simulink model "SF051A_SnsrOffsLrng"  (R2013b)
settings: Solver=FixedStepDiscrete  SolverMode=SingleTasking  StartTime=0.0  StopTime=1  FixedStep=0.002  RelTol=1e-3
values from neighbouring files (symbols this model uses):
  ARCHGLBPRM_10MILLISEC_SEC_F32 = DataDict.Constant    [SF051A_SnsrOffsLrng_DataDict.m]
  ARCHGLBPRM_2MILLISEC_SEC_F32 = DataDict.Constant    [SF051A_SnsrOffsLrng_DataDict.m]
  ARCHGLBPRM_2PI_ULS_F32 = DataDict.Constant    [SF051A_SnsrOffsLrng_DataDict.m]
  ARCHGLBPRM_FLOATZEROTHD_ULS_F32 = DataDict.Constant    [SF051A_SnsrOffsLrng_DataDict.m]
  ARCHGLBPRM_PIOVER180_ULS_F32 = DataDict.Constant    [SF051A_SnsrOffsLrng_DataDict.m]
  CNV100MICROSECTOSEC_SECPERCNT_F32 = DataDict.Constant    [SF051A_SnsrOffsLrng_DataDict.m]
  COVRAMTRXNIT_ULS_F32 = DataDict.Constant    [SF051A_SnsrOffsLrng_DataDict.m]
  HWAGHILIM_HWDEG_F32 = DataDict.Constant    [SF051A_SnsrOffsLrng_DataDict.m]
  HWAUTHYTHD_ULS_F32 = DataDict.Constant    [SF051A_SnsrOffsLrng_DataDict.m]
  HWTQLRNGSTSLRND_CNT_U08 = DataDict.Constant    [SF051A_SnsrOffsLrng_DataDict.m]
  HWTQLRNGSTSNEGOFFS_CNT_U08 = DataDict.Constant    [SF051A_SnsrOffsLrng_DataDict.m]
  HWTQLRNGSTSNOTLRND_CNT_U08 = DataDict.Constant    [SF051A_SnsrOffsLrng_DataDict.m]
  HWTQLRNGSTSPOSOFFS_CNT_U08 = DataDict.Constant    [SF051A_SnsrOffsLrng_DataDict.m]
  HWTQLRNGSTSZEROOFFS_CNT_U08 = DataDict.Constant    [SF051A_SnsrOffsLrng_DataDict.m]
  IDYMTRX_ULS_F32 = DataDict.Constant    [SF051A_SnsrOffsLrng_DataDict.m]
  IVS10MS_ULSPERSEC_F32 = DataDict.Constant    [SF051A_SnsrOffsLrng_DataDict.m]
  LRNGFILTICON_ULS_F32 = DataDict.Constant    [SF051A_SnsrOffsLrng_DataDict.m]
  ONE_ULS_F32 = DataDict.Constant    [SF051A_SnsrOffsLrng_DataDict.m]
  SnsrOffsLrnd = DataDict.NVM    [SF051A_SnsrOffsLrng_DataDict.m]
  SnsrOffsLrngFctEna = DataDict.Calibration    [SF051A_SnsrOffsLrng_DataDict.m]
  SnsrOffsLrngHwAgLrngDrvgDstThd = DataDict.Calibration    [SF051A_SnsrOffsLrng_DataDict.m]
  SnsrOffsLrngHwAgLrngEna = DataDict.Calibration    [SF051A_SnsrOffsLrng_DataDict.m]
  SnsrOffsLrngHwAgLrngHwVelThd = DataDict.Calibration    [SF051A_SnsrOffsLrng_DataDict.m]
  SnsrOffsLrngHwAgLrngSysTqThd = DataDict.Calibration    [SF051A_SnsrOffsLrng_DataDict.m]
  SnsrOffsLrngHwAgLrngSysTqThdMed = DataDict.Calibration    [SF051A_SnsrOffsLrng_DataDict.m]
  SnsrOffsLrngHwAgLrngSysTqThdTrustd = DataDict.Calibration    [SF051A_SnsrOffsLrng_DataDict.m]
  SnsrOffsLrngHwAgLrngSysTqThdWide = DataDict.Calibration    [SF051A_SnsrOffsLrng_DataDict.m]
  SnsrOffsLrngHwAgLrngTi = DataDict.Calibration    [SF051A_SnsrOffsLrng_DataDict.m]
  SnsrOffsLrngHwAgLrngVehSpdThd = DataDict.Calibration    [SF051A_SnsrOffsLrng_DataDict.m]
  SnsrOffsLrngHwAgLrngYawOffsDbnd = DataDict.Calibration    [SF051A_SnsrOffsLrng_DataDict.m]
  SnsrOffsLrngHwAgLrngYawRateThd = DataDict.Calibration    [SF051A_SnsrOffsLrng_DataDict.m]
  SnsrOffsLrngHwAgOffsLim = DataDict.Calibration    [SF051A_SnsrOffsLrng_DataDict.m]
  SnsrOffsLrngHwTqLrngEna = DataDict.Calibration    [SF051A_SnsrOffsLrng_DataDict.m]
  SnsrOffsLrngHwTqLrngEnaTiThd = DataDict.Calibration    [SF051A_SnsrOffsLrng_DataDict.m]
  SnsrOffsLrngHwTqLrngHwAgDbnd = DataDict.Calibration    [SF051A_SnsrOffsLrng_DataDict.m]
  SnsrOffsLrngHwTqLrngHwAgThd = DataDict.Calibration    [SF051A_SnsrOffsLrng_DataDict.m]
  SnsrOffsLrngHwTqLrngHwTqThd = DataDict.Calibration    [SF051A_SnsrOffsLrng_DataDict.m]
  SnsrOffsLrngHwTqLrngHwTqZeroOffsThd = DataDict.Calibration    [SF051A_SnsrOffsLrng_DataDict.m]
  SnsrOffsLrngHwTqLrngHwVelThd = DataDict.Calibration    [SF051A_SnsrOffsLrng_DataDict.m]
  SnsrOffsLrngHwTqLrngMeasTi = DataDict.Calibration    [SF051A_SnsrOffsLrng_DataDict.m]
  SnsrOffsLrngHwTqLrngMeasTiScar = DataDict.Calibration    [SF051A_SnsrOffsLrng_DataDict.m]
  SnsrOffsLrngHwTqLrngSampleImbThd1 = DataDict.Calibration    [SF051A_SnsrOffsLrng_DataDict.m]
  SnsrOffsLrngHwTqLrngSampleImbThd2 = DataDict.Calibration    [SF051A_SnsrOffsLrng_DataDict.m]
  SnsrOffsLrngHwTqLrngSampleThd1 = DataDict.Calibration    [SF051A_SnsrOffsLrng_DataDict.m]
  SnsrOffsLrngHwTqLrngSampleThd2 = DataDict.Calibration    [SF051A_SnsrOffsLrng_DataDict.m]
  SnsrOffsLrngHwTqLrngTiWghtCoeff = DataDict.Calibration    [SF051A_SnsrOffsLrng_DataDict.m]
  SnsrOffsLrngHwTqLrngVehSpdThd = DataDict.Calibration    [SF051A_SnsrOffsLrng_DataDict.m]
  SnsrOffsLrngHwTqOffsLim = DataDict.Calibration    [SF051A_SnsrOffsLrng_DataDict.m]
  SnsrOffsLrngSampleCntForHwTqLrngRst = DataDict.Calibration    [SF051A_SnsrOffsLrng_DataDict.m]
  SnsrOffsLrngTqInpDetnPwrEstimnThd = DataDict.Calibration    [SF051A_SnsrOffsLrng_DataDict.m]
  SnsrOffsLrngTqInpDetnSinGenrAmp = DataDict.Calibration    [SF051A_SnsrOffsLrng_DataDict.m]
  SnsrOffsLrngTqInpDetnSinGenrFrq = DataDict.Calibration    [SF051A_SnsrOffsLrng_DataDict.m]
  SnsrOffsLrngTqInpDetnStg1FilGain = DataDict.Calibration    [SF051A_SnsrOffsLrng_DataDict.m]
  SnsrOffsLrngTqInpDetnStg1WinSize = DataDict.Calibration    [SF051A_SnsrOffsLrng_DataDict.m]
  SnsrOffsLrngTqInpDetnStg2FilGainCen = DataDict.Calibration    [SF051A_SnsrOffsLrng_DataDict.m]
  SnsrOffsLrngTqInpDetnStg2FilGainDwn = DataDict.Calibration    [SF051A_SnsrOffsLrng_DataDict.m]
  SnsrOffsLrngTqInpDetnStg2FilGainUp = DataDict.Calibration    [SF051A_SnsrOffsLrng_DataDict.m]
  SnsrOffsLrngTqInpDetnStg2WinSize = DataDict.Calibration    [SF051A_SnsrOffsLrng_DataDict.m]
  SnsrOffsLrngYawLrngEna = DataDict.Calibration    [SF051A_SnsrOffsLrng_DataDict.m]
  SnsrOffsLrngYawLrngHwAgThd = DataDict.Calibration    [SF051A_SnsrOffsLrng_DataDict.m]
  SnsrOffsLrngYawLrngTi = DataDict.Calibration    [SF051A_SnsrOffsLrng_DataDict.m]
  SnsrOffsLrngYawLrngYawAThd = DataDict.Calibration    [SF051A_SnsrOffsLrng_DataDict.m]
  SnsrOffsLrngYawOffsFrshTiThd = DataDict.Calibration    [SF051A_SnsrOffsLrng_DataDict.m]
  SnsrOffsLrngYawRateOffsLim = DataDict.Calibration    [SF051A_SnsrOffsLrng_DataDict.m]
  SPDCNVN_MTRPERSECPERKPH_F32 = DataDict.Constant    [SF051A_SnsrOffsLrng_DataDict.m]
  SysGlbPrmSysTqRat = DataDict.ImprtdCal    [SF051A_SnsrOffsLrng_DataDict.m]
  TISTEP10MS_MINS_F32 = DataDict.Constant    [SF051A_SnsrOffsLrng_DataDict.m]
  TQINPDETNLOGGAIN_ULS_F32 = DataDict.Constant    [SF051A_SnsrOffsLrng_DataDict.m]
  YAWELPDTIHILIM_MINS_F32 = DataDict.Constant    [SF051A_SnsrOffsLrng_DataDict.m]
  YAWRATENOISE_VEHDEGPERSEC_F32 = DataDict.Constant    [SF051A_SnsrOffsLrng_DataDict.m]
  ZERO_ULS_F32 = DataDict.Constant    [SF051A_SnsrOffsLrng_DataDict.m]
  ZEROVECT_ULS_F32 = DataDict.Constant    [SF051A_SnsrOffsLrng_DataDict.m]
undefined symbols (not defined in the file or in its folder): NvmGetErrSts1
libraries: Fil x34, NxtrLim x20, FixdToFloat x17, FloatToFixd x16, simulink x12, NxtrAbslt x12, NxtrNvM x8, NxtrMath x3
(part 11 of 12)

== system SF051A_SnsrOffsLrng/SnsrOffsLrng/SnsrOffsLrngPer2/Enable_Function/POC/Learn/BiasEstimation_ValidityCheck/HwTqAvrg_Check ==
  note: SysTrq is the addition of the Driver's torque and the Assist torque
      | (in HwNm coordinates)
  note: SysTrqAVG is the average SysTrq during the time that the
      | Learning filters were enabled.
  note: TOCStatus
      | 0 = HwTrq NotLearned
      | 1 = Positive HwTrq Offset
      | 2 = Negative HwTrqOffset
      | 3 = Zero HwTrq Offset
      | 4 = HwTrq Offset Learned
  SysTqAvrg : Inport
  HwTqLrngSts : Inport  Port=2  OutDataTypeStr=uint8
  Constant : Constant  Value=SnsrOffsLrngHwAgLrngSysTqThdTrustd  OutDataTypeStr=single
  Constant1 : Constant  Value=SnsrOffsLrngHwAgLrngSysTqThdWide  OutDataTypeStr=single
  Constant2 : Constant  Value=SnsrOffsLrngHwAgLrngSysTqThdMed  OutDataTypeStr=single
  Display1 : DataStoreWrite  DataStoreName=dSnsrOffsLrngHwAgLrngSysTqUpThd
  Display2 : DataStoreWrite  DataStoreName=dSnsrOffsLrngHwAgLrngSysTqLoThd
  Display3 : DataStoreWrite  DataStoreName=dSnsrOffsLrngHwAgLrngSysTqVldt
  Logical Operator : Logic  AllPortsSameDT=off  OutDataTypeStr=boolean
  Merge_LowTh : Merge  Inputs=6
  Merge_UpTh : Merge  Inputs=6
  Relational Operator : RelationalOperator  Operator=<=  OutDataTypeStr=boolean
  Relational Operator1 : RelationalOperator  OutDataTypeStr=boolean
  Subsystem5 : Subsystem  Description=|  mask(Copyright Information){none=on}
      | Copyright info block.                                               
      |                                                                     
      | Place copyright information at the top of every subsystem in design.
      mask prompts: none "No parameters"
      mask help: Place copyright information at the top of every subsystem in design.
      mask Display:
      | NxtrConf = 'Nexteer Confidential';
      | 
      | sys = bdroot; %handle for the current model ("system")
      | first = get_param(sys,'Created');
      | first = first(end-3:end);  %year is last four digits
      | 
      | last = get_param(sys,'LastModifiedDate');
      | if isempty(last)
      |     last = datestr(now,'yyyy');
      | else
      |     last = last(end-3:end);
      | end
      | 
      | if strcmp(first,last)
      |     fprintf('%s -- Copyright %s Nexteer',NxtrConf,first)
      | else
      |     fprintf('%s -- %s%s- %s Nexteer',NxtrConf,char(169),first,last)
      | end
  Switch Case : SwitchCase  CaseConditions={0,1,2,3,4}
  Switch Case Action Subsystem : Subsystem  RequirementInfo="{'linktype_rmi_doors' '0000babd (/E-STEER Core/SubSystem Specifications/Application Functions/SF051A Sensor Offset Learning)' '#SF051A_146' 'true' 'REQ:  SF051A_146' '' } %GIDa_e88fd376_b621_43d8_82e5_da5b2ad99d04"  TreatAsAtomicUnit=on
  Switch Case Action Subsystem1 : Subsystem  RequirementInfo="{'linktype_rmi_doors' '0000babd (/E-STEER Core/SubSystem Specifications/Application Functions/SF051A Sensor Offset Learning)' '#SF051A_145' 'true' 'REQ:  SF051A_145' '' } %GIDa_07809d37_1ffe_4fb4_b852_393f01c2375c"  TreatAsAtomicUnit=on
  Switch Case Action Subsystem2 : Subsystem  RequirementInfo="{'linktype_rmi_doors' '0000babd (/E-STEER Core/SubSystem Specifications/Application Functions/SF051A Sensor Offset Learning)' '#SF051A_144' 'true' 'REQ:  SF051A_144' '' } %GIDa_dd268c2c_ea11_4446_9a40_dacfc2e25d53"  TreatAsAtomicUnit=on
  Switch Case Action Subsystem3 : Subsystem  RequirementInfo={'linktype_rmi_doors' '0000babd (/E-STEER Core/SubSystem Specifications/Application Functions/SF051A Sensor Offset Learning)' '#SF051A_143' 'true' 'REQ: SF051A_143' '' } %GIDa_217b07df_1d8f_435d_a8bd_62cab7965346  TreatAsAtomicUnit=on
  Switch Case Action Subsystem4 : Subsystem  RequirementInfo="{'linktype_rmi_doors' '0000babd (/E-STEER Core/SubSystem Specifications/Application Functions/SF051A Sensor Offset Learning)' '#SF051A_142' 'true' 'REQ:  SF051A_142' '' } %GIDa_01db2596_4f13_4ac9_b73b_dfc9e16a8861"  TreatAsAtomicUnit=on
  Switch Case Action Subsystem5 : Subsystem  TreatAsAtomicUnit=on
  TqVldFlg : Outport
  wires:
  HwTqLrngSts/1 -> Switch Case/1
  Switch Case Action Subsystem/1(UpTh) -> Merge_UpTh/1
  Merge_UpTh/1 -> Relational Operator/2, Display1/1
  Merge_LowTh/1 -> Display2/1, Relational Operator1/2
  Switch Case/2 -> Switch Case Action Subsystem1/Action
  Switch Case/3 -> Switch Case Action Subsystem2/Action
  Switch Case/4 -> Switch Case Action Subsystem3/Action
  Switch Case/5 -> Switch Case Action Subsystem4/Action
  Switch Case Action Subsystem1/1(UpTh) -> Merge_UpTh/2
  Switch Case Action Subsystem2/1(UpTh) -> Merge_UpTh/3
  Switch Case Action Subsystem3/1(UpTh) -> Merge_UpTh/4
  Switch Case Action Subsystem4/1(UpTh) -> Merge_UpTh/5
  Switch Case Action Subsystem/2(LowTh) -> Merge_LowTh/1
  Switch Case Action Subsystem1/2(LowTh) -> Merge_LowTh/2
  Switch Case Action Subsystem2/2(LowTh) -> Merge_LowTh/3
  Switch Case Action Subsystem3/2(LowTh) -> Merge_LowTh/4
  Switch Case Action Subsystem4/2(LowTh) -> Merge_LowTh/5
  Constant1/1 -> Switch Case Action Subsystem2/1(SysTqThdWide), Switch Case Action Subsystem5/1(SysTqThdWide), Switch Case Action Subsystem1/1(SysTqThdWide), Switch Case Action Subsystem/1(SysTqThdWide)
  Constant/1 -> Switch Case Action Subsystem4/1(SysTqThdTrustd)
  Constant2/1 -> Switch Case Action Subsystem3/1(SysTqThdMed)
  Switch Case/6 -> Switch Case Action Subsystem5/Action
  Switch Case/1 -> Switch Case Action Subsystem/Action
  Switch Case Action Subsystem5/1(UpTh) -> Merge_UpTh/6
  Switch Case Action Subsystem5/2(LowTh) -> Merge_LowTh/6
  SysTqAvrg/1 -> Relational Operator/1, Relational Operator1/1
  Relational Operator/1 -> Logical Operator/1
  Logical Operator/1 -> Display3/1, TqVldFlg/1
  Relational Operator1/1 -> Logical Operator/2

== system SF051A_SnsrOffsLrng/SnsrOffsLrng/SnsrOffsLrngPer2/Enable_Function/POC/Learn/BiasEstimation_ValidityCheck/Limit and Keep Learned Value ==
  HwPosBiasEstRaw : Inport
  Action Port : ActionPort  ActionType=then
  Constant : Constant  RequirementInfo={'linktype_rmi_doors' '0000babd (/E-STEER Core/SubSystem Specifications/Application Functions/SF051A Sensor Offset Learning)' '#SF051A_138' 'true' 'REQ: SF051A_138' '' } %GIDa_21289eda_9e85_4347_9687_653c781a611d  Value=ZERO_ULS_F32  OutDataTypeStr=single
      settings: AttributesFormatString=%<OutDataTypeStr>
  Constant1 : Constant  RequirementInfo="{'linktype_rmi_doors' '0000babd (/E-STEER Core/SubSystem Specifications/Application Functions/SF051A Sensor Offset Learning)' '#SF051A_140' 'true' 'REQ:  SF051A_140' '' } %GIDa_a6f07fad_f17c_4ace_8365_667990c14b30"  Value=SnsrOffsLrngHwAgOffsLim  OutDataTypeStr=single
  FloatToFixd_s16_f32 : FloatToFixd/FloatToFixd_s16_f32  Param1=10
  LimDyn_f32 : NxtrLim/LimDyn_f32  RequirementInfo="{'linktype_rmi_doors' '0000babd (/E-STEER Core/SubSystem Specifications/Application Functions/SF051A Sensor Offset Learning)' '#SF051A_140' 'true' 'REQ:  SF051A_140' '' } %GIDa_2915a7af_cb2e_4592_b132_f2e0d313b25c"
  NVM Ram : DataStoreWrite  RequirementInfo="{'linktype_rmi_doors' '0000babd (/E-STEER Core/SubSystem Specifications/Application Functions/SF051A Sensor Offset Learning)' '#SF051A_120' 'true' 'REQ: SF051A_120' '' ; 'linktype_rmi_doors' '0000babd (/E-STEER Core/SubSystem Specifications/Application Functions/SF051A Sensor Offset Learning)' '#SF051A_119' 'true' 'REQ:  SF051A_119' '' } %GIDa_c18d5963_4a3f_423e_af1b_c67d16260ba6"  DataStoreName=SnsrOffsLrnd  DataStoreElements=SnsrOffsLrnd.HwAgLrndTi#SnsrOffsLrnd.HwAgOffs
  Subsystem5 : Subsystem  Description=|  mask(Copyright Information){none=on}
      | Copyright info block.                                               
      |                                                                     
      | Place copyright information at the top of every subsystem in design.
      mask prompts: none "No parameters"
      mask help: Place copyright information at the top of every subsystem in design.
      mask Display:
      | NxtrConf = 'Nexteer Confidential';
      | 
      | sys = bdroot; %handle for the current model ("system")
      | first = get_param(sys,'Created');
      | first = first(end-3:end);  %year is last four digits
      | 
      | last = get_param(sys,'LastModifiedDate');
      | if isempty(last)
      |     last = datestr(now,'yyyy');
      | else
      |     last = last(end-3:end);
      | end
      | 
      | if strcmp(first,last)
      |     fprintf('%s -- Copyright %s Nexteer',NxtrConf,first)
      | else
      |     fprintf('%s -- %s%s- %s Nexteer',NxtrConf,char(169),first,last)
      | end
  Unary Minus : UnaryMinus  RequirementInfo="{'linktype_rmi_doors' '0000babd (/E-STEER Core/SubSystem Specifications/Application Functions/SF051A Sensor Offset Learning)' '#SF051A_140' 'true' 'REQ:  SF051A_140' '' } %GIDa_fa7a1a43_c58a_4d89_8cd2_8f38148a6033"
  wires:
  Constant/1 -> NVM Ram/1
  LimDyn_f32/1 -> FloatToFixd_s16_f32/1
  Unary Minus/1 -> LimDyn_f32/2
  Constant1/1 -> LimDyn_f32/3, Unary Minus/1
  HwPosBiasEstRaw/1 -> LimDyn_f32/1
  FloatToFixd_s16_f32/1 -> NVM Ram/2

== system SF051A_SnsrOffsLrng/SnsrOffsLrng/SnsrOffsLrngPer2/Enable_Function/POC/Learn/BiasEstimation_ValidityCheck/Reset_HwAgLrng ==
  note: Suggest coding as inline local function: void Reset_HwAg_Learning()
  note: Set HwAg Offlset learning filter back to the last good learned value written to NVM Ram.
      | Set elapsed learning time back to zero.
  note: Reset timer
  note: Reset filters
  Action Port : ActionPort  ActionType=elseif
  Constant : Constant  RequirementInfo="{'linktype_rmi_doors' '0000babd (/E-STEER Core/SubSystem Specifications/Application Functions/SF051A Sensor Offset Learning)' '#SF051A_139' 'true' 'REQ:  SF051A_139' '' } %GIDa_4560022c_466c_4507_b52b_9d9e5f5221da"  Value=ZERO_ULS_F32  OutDataTypeStr=single
      settings: AttributesFormatString=%<OutDataTypeStr>
  Constant1 : Constant  RequirementInfo="{'linktype_rmi_doors' '0000babd (/E-STEER Core/SubSystem Specifications/Application Functions/SF051A Sensor Offset Learning)' '#SF051A_139' 'true' 'REQ:  SF051A_139' '' } %GIDa_5e13df5a_3650_4084_aa1a_80989b1f2780"  Value=ZERO_ULS_F32  OutDataTypeStr=single
      settings: AttributesFormatString=%<OutDataTypeStr>
  Filter SV : DataStoreWrite  RequirementInfo="{'linktype_rmi_doors' '0000babd (/E-STEER Core/SubSystem Specifications/Application Functions/SF051A Sensor Offset Learning)' '#SF051A_139' 'true' 'REQ:  SF051A_139' '' } %GIDa_be755dd9_fcb9_4425_99f4_faf64e25047e"  DataStoreName=HwAgLrngFil1  DataStoreElements=HwAgLrngFil1.FilSt
  Filter SV1 : DataStoreWrite  RequirementInfo="{'linktype_rmi_doors' '0000babd (/E-STEER Core/SubSystem Specifications/Application Functions/SF051A Sensor Offset Learning)' '#SF051A_139' 'true' 'REQ:  SF051A_139' '' } %GIDa_db09f921_4b2f_4c4a_a571_f8085cef7377"  DataStoreName=HwAgLrngFil2  DataStoreElements=HwAgLrngFil2.FilSt
  Filter SV2 : DataStoreWrite  RequirementInfo="{'linktype_rmi_doors' '0000babd (/E-STEER Core/SubSystem Specifications/Application Functions/SF051A Sensor Offset Learning)' '#SF051A_139' 'true' 'REQ:  SF051A_139' '' } %GIDa_eca337dd_6526_4b71_a1b3_c946e62c85db"  DataStoreName=HwAgLrngSysTqFil1  DataStoreElements=HwAgLrngSysTqFil1.FilSt
  Filter SV3 : DataStoreWrite  RequirementInfo="{'linktype_rmi_doors' '0000babd (/E-STEER Core/SubSystem Specifications/Application Functions/SF051A Sensor Offset Learning)' '#SF051A_139' 'true' 'REQ:  SF051A_139' '' } %GIDa_b7490b1d_2567_4876_95c7_4a522d04e094"  DataStoreName=HwAgLrngSysTqFil2  DataStoreElements=HwAgLrngSysTqFil2.FilSt
  FixdToFloat_f32_s16 : FixdToFloat/FixdToFloat_f32_s16  RequirementInfo="{'linktype_rmi_doors' '0000babd (/E-STEER Core/SubSystem Specifications/Application Functions/SF051A Sensor Offset Learning)' '#SF051A_139' 'true' 'REQ:  SF051A_139' '' } %GIDa_07f227f4_e48d_450e_941a_caccc55d408c"  Param1=10
  FloatToFixd_s16_f1 : FloatToFixd/FloatToFixd_s16_f32  RequirementInfo="{'linktype_rmi_doors' '0000babd (/E-STEER Core/SubSystem Specifications/Application Functions/SF051A Sensor Offset Learning)' '#SF051A_139' 'true' 'REQ:  SF051A_139' '' } %GIDa_9f4cd521_c682_414e_8f7b_f4d8bb8d08d8"  Param1=4
  FloatToFixd_s16_f32 : FloatToFixd/FloatToFixd_s16_f32  RequirementInfo="{'linktype_rmi_doors' '0000babd (/E-STEER Core/SubSystem Specifications/Application Functions/SF051A Sensor Offset Learning)' '#SF051A_139' 'true' 'REQ:  SF051A_139' '' } %GIDa_eb1dd361_8662_488a_ae55_706cff78fefd"  Param1=5
  NVMRam_Read : DataStoreRead  RequirementInfo="{'linktype_rmi_doors' '0000babd (/E-STEER Core/SubSystem Specifications/Application Functions/SF051A Sensor Offset Learning)' '#SF051A_139' 'true' 'REQ:  SF051A_139' '' } %GIDa_177ac313_4fc5_4d7a_9c86_b1caf788b8ab"  DataStoreName=SnsrOffsLrnd  DataStoreElements=SnsrOffsLrnd.YawRateOffs
  Read NVM Ram : DataStoreRead  RequirementInfo="{'linktype_rmi_doors' '0000babd (/E-STEER Core/SubSystem Specifications/Application Functions/SF051A Sensor Offset Learning)' '#SF051A_139' 'true' 'REQ:  SF051A_139' '' } %GIDa_cc646748_aa1c_414f_b217_a4a1e7ec684c"  DataStoreName=SnsrOffsLrnd  DataStoreElements=SnsrOffsLrnd.HwAgOffs
  Subsystem5 : Subsystem  Description=|  mask(Copyright Information){none=on}
      | Copyright info block.                                               
      |                                                                     
      | Place copyright information at the top of every subsystem in design.
      mask prompts: none "No parameters"
      mask help: Place copyright information at the top of every subsystem in design.
      mask Display:
      | NxtrConf = 'Nexteer Confidential';
      | 
      | sys = bdroot; %handle for the current model ("system")
      | first = get_param(sys,'Created');
      | first = first(end-3:end);  %year is last four digits
      | 
      | last = get_param(sys,'LastModifiedDate');
      | if isempty(last)
      |     last = datestr(now,'yyyy');
      | else
      |     last = last(end-3:end);
      | end
      | 
      | if strcmp(first,last)
      |     fprintf('%s -- Copyright %s Nexteer',NxtrConf,first)
      | else
      |     fprintf('%s -- %s%s- %s Nexteer',NxtrConf,char(169),first,last)
      | end
  Update Reference : DataStoreWrite  RequirementInfo="{'linktype_rmi_doors' '0000babd (/E-STEER Core/SubSystem Specifications/Application Functions/SF051A Sensor Offset Learning)' '#SF051A_139' 'true' 'REQ:  SF051A_139' '' } %GIDa_1dfc11a1_5f56_44a1_bae8_84f200f7324d"  DataStoreName=SnsrOffsLrnd  DataStoreElements=SnsrOffsLrnd.HwAgLrngYawOffsRef
  Write NVM Ram : DataStoreWrite  RequirementInfo="{'linktype_rmi_doors' '0000babd (/E-STEER Core/SubSystem Specifications/Application Functions/SF051A Sensor Offset Learning)' '#SF051A_139' 'true' 'REQ:  SF051A_139' '' } %GIDa_39324f37_a93b_47b6_9df3_ec328393f6b7"  DataStoreName=SnsrOffsLrnd  DataStoreElements=SnsrOffsLrnd.HwAgLrndTi
  Write NVM Ram1 : DataStoreWrite  RequirementInfo="{'linktype_rmi_doors' '0000babd (/E-STEER Core/SubSystem Specifications/Application Functions/SF051A Sensor Offset Learning)' '#SF051A_139' 'true' 'REQ:  SF051A_139' '' } %GIDa_e39abcc7_e566_46cb_a681_dee0ec267987"  DataStoreName=SnsrOffsLrnd  DataStoreElements=SnsrOffsLrnd.HwAgLrngHwAgFilSt#SnsrOffsLrnd.HwAgLrngSysTqFilSt
  wires:
  Constant/1 -> Write NVM Ram/1
  NVMRam_Read/1 -> Update Reference/1
  Read NVM Ram/1 -> FixdToFloat_f32_s16/1
  Constant1/1 -> Filter SV3/1, Filter SV2/1, FloatToFixd_s16_f32/1
  FixdToFloat_f32_s16/1 -> Filter SV/1, FloatToFixd_s16_f1/1, Filter SV1/1
  FloatToFixd_s16_f1/1 -> Write NVM Ram1/1
  FloatToFixd_s16_f32/1 -> Write NVM Ram1/2

== system SF051A_SnsrOffsLrng/SnsrOffsLrng/SnsrOffsLrngPer2/Enable_Function/POC/Learn/BiasEstimation_ValidityCheck/Subsystem5 ==

== system SF051A_SnsrOffsLrng/SnsrOffsLrng/SnsrOffsLrngPer2/Enable_Function/POC/Learn/BiasEstimation_ValidityCheck/Time_Check ==
  ElpsdTi : Inport  RequirementInfo="{'linktype_rmi_doors' '0000babd (/E-STEER Core/SubSystem Specifications/Application Functions/SF051A Sensor Offset Learning)' '#SF051A_118' 'true' 'REQ:  SF051A_118' '' } %GIDa_ec54a004_f423_4b2c_b946_d1b5b6921296"
  Constant1 : Constant  RequirementInfo="{'linktype_rmi_doors' '0000babd (/E-STEER Core/SubSystem Specifications/Application Functions/SF051A Sensor Offset Learning)' '#SF051A_122' 'true' 'REQ: SF051A_122' '' ; 'linktype_rmi_doors' '0000babd (/E-STEER Core/SubSystem Specifications/Application Functions/SF051A Sensor Offset Learning)' '#SF051A_117' 'true' 'REQ:  SF051A_117' '' } %GIDa_c643d9d6_48fd_4a4d_910f_6142205684cf"  Value=SnsrOffsLrngHwAgLrngTi
  Display1 : DataStoreWrite  DataStoreName=dSnsrOffsLrngHwAgLrngTiVldt
  LimStat_f32 : NxtrLim/LimStat_f32  RequirementInfo="{'linktype_rmi_doors' '0000babd (/E-STEER Core/SubSystem Specifications/Application Functions/SF051A Sensor Offset Learning)' '#SF051A_118' 'true' 'REQ:  SF051A_118' '' } %GIDa_ad840ae8_cbbf_4568_afc2_9c7d4c9a189f"  LoLim=ZERO_ULS_F32  HiLim=SnsrOffsLrngHwAgLrngTi
      settings: AttributesFormatString=|
      | Low Limit: %<LoLim>
      | High Limit:%<HiLim>
  Relational Operator1 : RelationalOperator  RequirementInfo="{'linktype_rmi_doors' '0000babd (/E-STEER Core/SubSystem Specifications/Application Functions/SF051A Sensor Offset Learning)' '#SF051A_117' 'true' 'REQ:  SF051A_117' '' } %GIDa_e756bea4_804a_407e_bb48_f5c0006da0a9"  OutDataTypeStr=boolean
  Subsystem5 : Subsystem  Description=|  mask(Copyright Information){none=on}
      | Copyright info block.                                               
      |                                                                     
      | Place copyright information at the top of every subsystem in design.
      mask prompts: none "No parameters"
      mask help: Place copyright information at the top of every subsystem in design.
      mask Display:
      | NxtrConf = 'Nexteer Confidential';
      | 
      | sys = bdroot; %handle for the current model ("system")
      | first = get_param(sys,'Created');
      | first = first(end-3:end);  %year is last four digits
      | 
      | last = get_param(sys,'LastModifiedDate');
      | if isempty(last)
      |     last = datestr(now,'yyyy');
      | else
      |     last = last(end-3:end);
      | end
      | 
      | if strcmp(first,last)
      |     fprintf('%s -- Copyright %s Nexteer',NxtrConf,first)
      | else
      |     fprintf('%s -- %s%s- %s Nexteer',NxtrConf,char(169),first,last)
      | end
  Write NVMRam : DataStoreWrite  RequirementInfo="{'linktype_rmi_doors' '0000babd (/E-STEER Core/SubSystem Specifications/Application Functions/SF051A Sensor Offset Learning)' '#SF051A_120' 'true' 'REQ:  SF051A_120' '' ; 'linktype_rmi_doors' '0000babd (/E-STEER Core/SubSystem Specifications/Application Functions/SF051A Sensor Offset Learning)' '#SF051A_119' 'true' 'REQ:  SF051A_119' '' ; 'linktype_rmi_doors' '0000babd (/E-STEER Core/SubSystem Specifications/Application Functions/SF051A Sensor Offset Learning)' '#SF051A_118' 'true' 'REQ:  SF051A_118' '' } %GIDa_6fdf401b_98e4_4250_8664_c2ed6dbc601a"  DataStoreName=SnsrOffsLrnd  DataStoreElements=SnsrOffsLrnd.HwAgLrndTi
  TiVldFlg : Outport
  wires:
  ElpsdTi/1 -> LimStat_f32/1, Relational Operator1/1  "ElpsdTi"
  LimStat_f32/1 -> Write NVMRam/1
  Constant1/1 -> Relational Operator1/2
  Relational Operator1/1 -> Display1/1, TiVldFlg/1

== system SF051A_SnsrOffsLrng/SnsrOffsLrng/SnsrOffsLrngPer2/Enable_Function/POC/Learn/LPFs/Subsystem5 ==

== system SF051A_SnsrOffsLrng/SnsrOffsLrng/SnsrOffsLrngPer2/Enable_Function/POC/Learning Conditions/DrivingStraight/Subsystem5 ==

== system SF051A_SnsrOffsLrng/SnsrOffsLrng/SnsrOffsLrngPer2/Enable_Function/POC/Learning Conditions/NotDrivingStraight/Subsystem5 ==

== system SF051A_SnsrOffsLrng/SnsrOffsLrng/SnsrOffsLrngPer2/Enable_Function/YOC/Learn/Do nothing/Subsystem5 ==

== system SF051A_SnsrOffsLrng/SnsrOffsLrng/SnsrOffsLrngPer2/Enable_Function/YOC/Learn/Filter For Learning/Subsystem5 ==

== system SF051A_SnsrOffsLrng/SnsrOffsLrng/SnsrOffsLrngPer2/Enable_Function/YOC/Learn/Update NVM RAM/Subsystem5 ==

== system SF051A_SnsrOffsLrng/SnsrOffsLrng/SnsrOffsLrngPer1/EnableLearning/Perform_TqInpDetn/Enable_PreProcessing/Preprocessing/Do nothing/Subsystem5 ==

== system SF051A_SnsrOffsLrng/SnsrOffsLrng/SnsrOffsLrngPer1/EnableLearning/Perform_TqInpDetn/Enable_PreProcessing/Preprocessing/General_Goertzel/Goertzel_Part1_1 ==
  note: s(n-2)
  note: Suggested Coding:  This can be an inline local function.  Simulink limitations prevent modeling it that way, so this block
      | is replicated multiple times throughout the component model.
  X0 : Inport
  FilGain : Inport  Port=2
  S2 : Inport  Port=3
  S1 : Inport  Port=4
  " Product1" : Product  Inputs=**
  Add1 : Sum  Inputs=++-
  Subsystem5 : Subsystem  Description=|  mask(Copyright Information){none=on}
      | Copyright info block.                                               
      |                                                                     
      | Place copyright information at the top of every subsystem in design.
      mask prompts: none "No parameters"
      mask help: Place copyright information at the top of every subsystem in design.
      mask Display:
      | NxtrConf = 'Nexteer Confidential';
      | 
      | sys = bdroot; %handle for the current model ("system")
      | first = get_param(sys,'Created');
      | first = first(end-3:end);  %year is last four digits
      | 
      | last = get_param(sys,'LastModifiedDate');
      | if isempty(last)
      |     last = datestr(now,'yyyy');
      | else
      |     last = last(end-3:end);
      | end
      | 
      | if strcmp(first,last)
      |     fprintf('%s -- Copyright %s Nexteer',NxtrConf,first)
      | else
      |     fprintf('%s -- %s%s- %s Nexteer',NxtrConf,char(169),first,last)
      | end
  S0 : Outport
  wires:
  Add1/1 -> S0/1
  " Product1"/1 -> Add1/2
  S2/1 -> Add1/3
  FilGain/1 -> " Product1"/1
  X0/1 -> Add1/1
  S1/1 -> " Product1"/2

== system SF051A_SnsrOffsLrng/SnsrOffsLrng/SnsrOffsLrngPer1/EnableLearning/Perform_TqInpDetn/Enable_PreProcessing/Preprocessing/General_Goertzel/Goertzel_Part1_2 ==
  note: s(n-2)
  note: Suggested Coding:  This can be an inline local function.  Simulink limitations prevent modeling it that way, so this block
      | is replicated multiple times throughout the component model.
  X0 : Inport
  FilGain : Inport  Port=2
  S2 : Inport  Port=3
  S1 : Inport  Port=4
  " Product1" : Product  Inputs=**
  Add1 : Sum  Inputs=++-
  Subsystem5 : Subsystem  Description=|  mask(Copyright Information){none=on}
      | Copyright info block.                                               
      |                                                                     
      | Place copyright information at the top of every subsystem in design.
      mask prompts: none "No parameters"
      mask help: Place copyright information at the top of every subsystem in design.
      mask Display:
      | NxtrConf = 'Nexteer Confidential';
      | 
      | sys = bdroot; %handle for the current model ("system")
      | first = get_param(sys,'Created');
      | first = first(end-3:end);  %year is last four digits
      | 
      | last = get_param(sys,'LastModifiedDate');
      | if isempty(last)
      |     last = datestr(now,'yyyy');
      | else
      |     last = last(end-3:end);
      | end
      | 
      | if strcmp(first,last)
      |     fprintf('%s -- Copyright %s Nexteer',NxtrConf,first)
      | else
      |     fprintf('%s -- %s%s- %s Nexteer',NxtrConf,char(169),first,last)
      | end
  S0 : Outport
  wires:
  Add1/1 -> S0/1
  " Product1"/1 -> Add1/2
  S2/1 -> Add1/3
  FilGain/1 -> " Product1"/1
  X0/1 -> Add1/1
  S1/1 -> " Product1"/2

== system SF051A_SnsrOffsLrng/SnsrOffsLrng/SnsrOffsLrngPer1/EnableLearning/Perform_TqInpDetn/Enable_PreProcessing/Preprocessing/General_Goertzel/Goertzel_Part1_3 ==
  note: s(n-2)
  note: Suggested Coding:  This can be an inline local function.  Simulink limitations prevent modeling it that way, so this block
      | is replicated multiple times throughout the component model.
  X0 : Inport
  FilGain : Inport  Port=2
  S2 : Inport  Port=3
  S1 : Inport  Port=4
  " Product1" : Product  Inputs=**
  Add1 : Sum  Inputs=++-
  Subsystem5 : Subsystem  Description=|  mask(Copyright Information){none=on}
      | Copyright info block.                                               
      |                                                                     
      | Place copyright information at the top of every subsystem in design.
      mask prompts: none "No parameters"
      mask help: Place copyright information at the top of every subsystem in design.
      mask Display:
      | NxtrConf = 'Nexteer Confidential';
      | 
      | sys = bdroot; %handle for the current model ("system")
      | first = get_param(sys,'Created');
      | first = first(end-3:end);  %year is last four digits
      | 
      | last = get_param(sys,'LastModifiedDate');
      | if isempty(last)
      |     last = datestr(now,'yyyy');
      | else
      |     last = last(end-3:end);
      | end
      | 
      | if strcmp(first,last)
      |     fprintf('%s -- Copyright %s Nexteer',NxtrConf,first)
      | else
      |     fprintf('%s -- %s%s- %s Nexteer',NxtrConf,char(169),first,last)
      | end
  S0 : Outport
  wires:
  Add1/1 -> S0/1
  " Product1"/1 -> Add1/2
  S2/1 -> Add1/3
  FilGain/1 -> " Product1"/1
  X0/1 -> Add1/1
  S1/1 -> " Product1"/2

== system SF051A_SnsrOffsLrng/SnsrOffsLrng/SnsrOffsLrngPer1/EnableLearning/Perform_TqInpDetn/Enable_PreProcessing/Preprocessing/General_Goertzel/Subsystem5 ==

== system SF051A_SnsrOffsLrng/SnsrOffsLrng/SnsrOffsLrngPer1/EnableLearning/Perform_TqInpDetn/Enable_PreProcessing/Preprocessing/NewOut_ResetCntr/Goertzel_Part2_1 ==
  note: abs(y(n))^2
  note: Suggested Coding:  This can be an inline local function.  Simulink limitations prevent modeling it that way, so this block
      | is replicated multiple times throughout the component model.
  note: s^2(n)
  note: s^2(n-1)
  note: s(n-1)
  note: In the academic definition of the goertzel algorithm this block would have a complex calculation.
      | Since we are only interested in the magnitude, the following is an implementation that only need real calculations.
  S0 : Inport
  S1 : Inport  Port=2
  FilGain : Inport  Port=3
  " Product5" : Product  Inputs=**
  Product2 : Product  Inputs=**
  Product3 : Product  Inputs=**
  Product4 : Product  Inputs=**
  Subsystem5 : Subsystem  Description=|  mask(Copyright Information){none=on}
      | Copyright info block.                                               
      |                                                                     
      | Place copyright information at the top of every subsystem in design.
      mask prompts: none "No parameters"
      mask help: Place copyright information at the top of every subsystem in design.
      mask Display:
      | NxtrConf = 'Nexteer Confidential';
      | 
      | sys = bdroot; %handle for the current model ("system")
      | first = get_param(sys,'Created');
      | first = first(end-3:end);  %year is last four digits
      | 
      | last = get_param(sys,'LastModifiedDate');
      | if isempty(last)
      |     last = datestr(now,'yyyy');
      | else
      |     last = last(end-3:end);
      | end
      | 
      | if strcmp(first,last)
      |     fprintf('%s -- Copyright %s Nexteer',NxtrConf,first)
      | else
      |     fprintf('%s -- %s%s- %s Nexteer',NxtrConf,char(169),first,last)
      | end
  add : Sum  Inputs=++-
  MagnSq : Outport
  wires:
  FilGain/1 -> " Product5"/2
  add/1 -> MagnSq/1
  Product2/1 -> add/1  "FiltSt0Sq_Uls_T_f32"
  Product3/1 -> add/2  "FiltSt1Sq_Uls_T_f32"
  Product4/1 -> " Product5"/1
  " Product5"/1 -> add/3  "FiltSt0St1_Uls_T_f32"
  S1/1 -> Product3/2, Product3/1, Product4/2
  S0/1 -> Product4/1, Product2/2, Product2/1

== system SF051A_SnsrOffsLrng/SnsrOffsLrng/SnsrOffsLrngPer1/EnableLearning/Perform_TqInpDetn/Enable_PreProcessing/Preprocessing/NewOut_ResetCntr/Goertzel_Part2_2 ==
  note: abs(y(n))^2
  note: Suggested Coding:  This can be an inline local function.  Simulink limitations prevent modeling it that way, so this block
      | is replicated multiple times throughout the component model.
  note: s^2(n)
  note: s^2(n-1)
  note: s(n-1)
  note: In the academic definition of the goertzel algorithm this block would have a complex calculation.
      | Since we are only interested in the magnitude, the following is an implementation that only need real calculations.
  S0 : Inport
  S1 : Inport  Port=2
  FilGain : Inport  Port=3
  " Product5" : Product  Inputs=**
  Product2 : Product  Inputs=**
  Product3 : Product  Inputs=**
  Product4 : Product  Inputs=**
  Subsystem5 : Subsystem  Description=|  mask(Copyright Information){none=on}
      | Copyright info block.                                               
      |                                                                     
      | Place copyright information at the top of every subsystem in design.
      mask prompts: none "No parameters"
      mask help: Place copyright information at the top of every subsystem in design.
      mask Display:
      | NxtrConf = 'Nexteer Confidential';
      | 
      | sys = bdroot; %handle for the current model ("system")
      | first = get_param(sys,'Created');
      | first = first(end-3:end);  %year is last four digits
      | 
      | last = get_param(sys,'LastModifiedDate');
      | if isempty(last)
      |     last = datestr(now,'yyyy');
      | else
      |     last = last(end-3:end);
      | end
      | 
      | if strcmp(first,last)
      |     fprintf('%s -- Copyright %s Nexteer',NxtrConf,first)
      | else
      |     fprintf('%s -- %s%s- %s Nexteer',NxtrConf,char(169),first,last)
      | end
  add : Sum  Inputs=++-
  MagnSq : Outport
  wires:
  FilGain/1 -> " Product5"/2
  add/1 -> MagnSq/1
  Product2/1 -> add/1  "FiltSt0Sq_Uls_T_f32"
  Product3/1 -> add/2  "FiltSt1Sq_Uls_T_f32"
  Product4/1 -> " Product5"/1
  " Product5"/1 -> add/3  "FiltSt0St1_Uls_T_f32"
  S1/1 -> Product3/2, Product3/1, Product4/2
  S0/1 -> Product4/1, Product2/2, Product2/1

== system SF051A_SnsrOffsLrng/SnsrOffsLrng/SnsrOffsLrngPer1/EnableLearning/Perform_TqInpDetn/Enable_PreProcessing/Preprocessing/NewOut_ResetCntr/Goertzel_Part2_3 ==
  note: abs(y(n))^2
  note: Suggested Coding:  This can be an inline local function.  Simulink limitations prevent modeling it that way, so this block
      | is replicated multiple times throughout the component model.
  note: s^2(n)
  note: s^2(n-1)
  note: s(n-1)
  note: In the academic definition of the goertzel algorithm this block would have a complex calculation.
      | Since we are only interested in the magnitude, the following is an implementation that only need real calculations.
  S0 : Inport
  S1 : Inport  Port=2
  FilGain : Inport  Port=3
  " Product5" : Product  Inputs=**
  Product2 : Product  Inputs=**
  Product3 : Product  Inputs=**
  Product4 : Product  Inputs=**
  Subsystem5 : Subsystem  Description=|  mask(Copyright Information){none=on}
      | Copyright info block.                                               
      |                                                                     
      | Place copyright information at the top of every subsystem in design.
      mask prompts: none "No parameters"
      mask help: Place copyright information at the top of every subsystem in design.
      mask Display:
      | NxtrConf = 'Nexteer Confidential';
      | 
      | sys = bdroot; %handle for the current model ("system")
      | first = get_param(sys,'Created');
      | first = first(end-3:end);  %year is last four digits
      | 
      | last = get_param(sys,'LastModifiedDate');
      | if isempty(last)
      |     last = datestr(now,'yyyy');
      | else
      |     last = last(end-3:end);
      | end
      | 
      | if strcmp(first,last)
      |     fprintf('%s -- Copyright %s Nexteer',NxtrConf,first)
      | else
      |     fprintf('%s -- %s%s- %s Nexteer',NxtrConf,char(169),first,last)
      | end
  add : Sum  Inputs=++-
  MagnSq : Outport
  wires:
  FilGain/1 -> " Product5"/2
  add/1 -> MagnSq/1
  Product2/1 -> add/1  "FiltSt0Sq_Uls_T_f32"
  Product3/1 -> add/2  "FiltSt1Sq_Uls_T_f32"
  Product4/1 -> " Product5"/1
  " Product5"/1 -> add/3  "FiltSt0St1_Uls_T_f32"
  S1/1 -> Product3/2, Product3/1, Product4/2
  S0/1 -> Product4/1, Product2/2, Product2/1

== system SF051A_SnsrOffsLrng/SnsrOffsLrng/SnsrOffsLrngPer1/EnableLearning/Perform_TqInpDetn/Enable_PreProcessing/Preprocessing/NewOut_ResetCntr/Subsystem5 ==

== system SF051A_SnsrOffsLrng/SnsrOffsLrng/SnsrOffsLrngPer1/EnableLearning/Perform_TqInpDetn/Enable_PreProcessing/Preprocessing/PrevOut_NoReset/Subsystem5 ==

== system SF051A_SnsrOffsLrng/SnsrOffsLrng/SnsrOffsLrngPer1/EnableLearning/Perform_TqInpDetn/Enable_PreProcessing/Preprocessing/SampleCounter/Subsystem5 ==

== system SF051A_SnsrOffsLrng/SnsrOffsLrng/SnsrOffsLrngPer1/EnableLearning/Perform_TqInpDetn/Enable_PreProcessing/Preprocessing/Sliding_Goertzel_ver001/SinGen ==
  note: This generates a sinusoidal command for a given frequency and fixed amplitude.  Based on logic found in SF043A, but simplified because
      | the frequency and amplitude values are just calibrations for this component.
  Add : Sum
  Angle_Wrapper : Subsystem
  Constant : Constant  Value=SnsrOffsLrngTqInpDetnSinGenrFrq
  Constant4 : Constant  Value=SnsrOffsLrngTqInpDetnSinGenrAmp
  Convert_To_Radians : Subsystem  TreatAsAtomicUnit=on
  Data Store Read : DataStoreRead  DataStoreName=TqInpDetnSinGenrAg
  Data Store Write : DataStoreWrite  DataStoreName=TqInpDetnSinGenrAg
  Product2 : Product  OutDataTypeStr=single  RndMeth=Zero
  Sin_f32 : NxtrMath/Sin_f32  SFunctionSpec=single y1 = Sin_f32(single u1)
      settings: AttributesFormatString=%<MaskType>
  Subsystem5 : Subsystem  Description=|  mask(Copyright Information){none=on}
      | Copyright info block.                                               
      |                                                                     
      | Place copyright information at the top of every subsystem in design.
      mask prompts: none "No parameters"
      mask help: Place copyright information at the top of every subsystem in design.
      mask Display:
      | NxtrConf = 'Nexteer Confidential';
      | 
      | sys = bdroot; %handle for the current model ("system")
      | first = get_param(sys,'Created');
      | first = first(end-3:end);  %year is last four digits
      | 
      | last = get_param(sys,'LastModifiedDate');
      | if isempty(last)
      |     last = datestr(now,'yyyy');
      | else
      |     last = last(end-3:end);
      | end
      | 
      | if strcmp(first,last)
      |     fprintf('%s -- Copyright %s Nexteer',NxtrConf,first)
      | else
      |     fprintf('%s -- %s%s- %s Nexteer',NxtrConf,char(169),first,last)
      | end
  TqOscCmd : Outport
  wires:
  Sin_f32/1 -> Product2/2
  Product2/1 -> TqOscCmd/1
  Angle_Wrapper/1(AgOut) -> Sin_f32/1, Data Store Write/1
  Add/1 -> Angle_Wrapper/1(AgIn)
  Constant4/1 -> Product2/1
  Constant/1 -> Convert_To_Radians/1(Freq)
  Convert_To_Radians/1(PhaAgStep) -> Add/1
  Data Store Read/1 -> Add/2

== system SF051A_SnsrOffsLrng/SnsrOffsLrng/SnsrOffsLrngPer1/EnableLearning/Perform_TqInpDetn/Enable_PreProcessing/Preprocessing/Sliding_Goertzel_ver001/SlidingGoertzel ==
  note: Limit to prevent log(0) = -inf
  note: Conversion to dB
  note: NOTE: Cal.EngMin = 1 to prevent divide-by-zero.
  HwTq : Inport
  Calculate_Magnitude : Subsystem
  Constant1 : Constant  Value=SnsrOffsLrngTqInpDetnStg1WinSize
  Constant2 : Constant  Value=TQINPDETNLOGGAIN_ULS_F32
  Data Type Conversion : DataTypeConversion  OutDataTypeStr=single
  Divide : Product  Inputs=*/
  LimStat_f32 : NxtrLim/LimStat_f32  LoLim=TQINPDETNLOGINPLOLIM_ULS_F32  HiLim=TQINPDETNLOGINPHILIM_ULS_F32
      settings: AttributesFormatString=|
      | Low Limit: %<LoLim>
      | High Limit:%<HiLim>
  Math Function1 : Math  Operator=log10  OutputSignalType=real  SaturateOnIntegerOverflow=on
  Product : Product
  Product1 : Product
  Sliding_Input : Subsystem
  Subsystem5 : Subsystem  Description=|  mask(Copyright Information){none=on}
      | Copyright info block.                                               
      |                                                                     
      | Place copyright information at the top of every subsystem in design.
      mask prompts: none "No parameters"
      mask help: Place copyright information at the top of every subsystem in design.
      mask Display:
      | NxtrConf = 'Nexteer Confidential';
      | 
      | sys = bdroot; %handle for the current model ("system")
      | first = get_param(sys,'Created');
      | first = first(end-3:end);  %year is last four digits
      | 
      | last = get_param(sys,'LastModifiedDate');
      | if isempty(last)
      |     last = datestr(now,'yyyy');
      | else
      |     last = last(end-3:end);
      | end
      | 
      | if strcmp(first,last)
      |     fprintf('%s -- Copyright %s Nexteer',NxtrConf,first)
      | else
      |     fprintf('%s -- %s%s- %s Nexteer',NxtrConf,char(169),first,last)
      | end
  Stg1Outp : Outport
  wires:
  Math Function1/1 -> Product1/1
  Product1/1 -> Stg1Outp/1
  HwTq/1 -> Sliding_Input/1(HwTq)
  Sliding_Input/1(x_n) -> Calculate_Magnitude/1(x_n)
  Calculate_Magnitude/1(MgnSq) -> Divide/1
  Product/1 -> Data Type Conversion/1
  Divide/1 -> LimStat_f32/1
  Constant1/1 -> Product/2, Product/1
  Data Type Conversion/1 -> Divide/2
  Constant2/1 -> Product1/2
  LimStat_f32/1 -> Math Function1/1

== system SF051A_SnsrOffsLrng/SnsrOffsLrng/SnsrOffsLrngPer1/EnableLearning/Perform_TqInpDetn/Enable_PreProcessing/Preprocessing/Sliding_Goertzel_ver001/Subsystem5 ==

== system SF051A_SnsrOffsLrng/SnsrOffsLrng/SnsrOffsLrngPer1/Learning/ValidityCheck/DecideOutputs/Pos//Neg//Zero Offset Status Selector/1_Positive HwTrq Offset/Subsystem5 ==

== system SF051A_SnsrOffsLrng/SnsrOffsLrng/SnsrOffsLrngPer1/Learning/ValidityCheck/DecideOutputs/Pos//Neg//Zero Offset Status Selector/2_Negative HwTrq Offset/Subsystem5 ==

== system SF051A_SnsrOffsLrng/SnsrOffsLrng/SnsrOffsLrngPer1/Learning/ValidityCheck/DecideOutputs/Pos//Neg//Zero Offset Status Selector/3_Zero HwTrq Offset/Subsystem5 ==

== system SF051A_SnsrOffsLrng/SnsrOffsLrng/SnsrOffsLrngPer2/Enable_Function/POC/Learn/BiasEstimation_ValidityCheck/Do nothing/Subsystem1 ==

== system SF051A_SnsrOffsLrng/SnsrOffsLrng/SnsrOffsLrngPer2/Enable_Function/POC/Learn/BiasEstimation_ValidityCheck/HwTqAvrg_Check/Subsystem5 ==

== system SF051A_SnsrOffsLrng/SnsrOffsLrng/SnsrOffsLrngPer2/Enable_Function/POC/Learn/BiasEstimation_ValidityCheck/HwTqAvrg_Check/Switch Case Action Subsystem ==
  SysTqThdWide : Inport
  Action Port : ActionPort  ActionType=case
  Gain : Gain  Gain=-1
  Subsystem5 : Subsystem  Description=|  mask(Copyright Information){none=on}
      | Copyright info block.                                               
      |                                                                     
      | Place copyright information at the top of every subsystem in design.
      mask prompts: none "No parameters"
      mask help: Place copyright information at the top of every subsystem in design.
      mask Display:
      | NxtrConf = 'Nexteer Confidential';
      | 
      | sys = bdroot; %handle for the current model ("system")
      | first = get_param(sys,'Created');
      | first = first(end-3:end);  %year is last four digits
      | 
      | last = get_param(sys,'LastModifiedDate');
      | if isempty(last)
      |     last = datestr(now,'yyyy');
      | else
      |     last = last(end-3:end);
      | end
      | 
      | if strcmp(first,last)
      |     fprintf('%s -- Copyright %s Nexteer',NxtrConf,first)
      | else
      |     fprintf('%s -- %s%s- %s Nexteer',NxtrConf,char(169),first,last)
      | end
  UpTh : Outport
  LowTh : Outport  Port=2
  wires:
  SysTqThdWide/1 -> Gain/1, UpTh/1
  Gain/1 -> LowTh/1

== system SF051A_SnsrOffsLrng/SnsrOffsLrng/SnsrOffsLrngPer2/Enable_Function/POC/Learn/BiasEstimation_ValidityCheck/HwTqAvrg_Check/Switch Case Action Subsystem1 ==
  SysTqThdWide : Inport
  Action Port : ActionPort  ActionType=case
  Constant : Constant  Value=ZERO_ULS_F32  OutDataTypeStr=single
      settings: AttributesFormatString=%<OutDataTypeStr>
  Subsystem5 : Subsystem  Description=|  mask(Copyright Information){none=on}
      | Copyright info block.                                               
      |                                                                     
      | Place copyright information at the top of every subsystem in design.
      mask prompts: none "No parameters"
      mask help: Place copyright information at the top of every subsystem in design.
      mask Display:
      | NxtrConf = 'Nexteer Confidential';
      | 
      | sys = bdroot; %handle for the current model ("system")
      | first = get_param(sys,'Created');
      | first = first(end-3:end);  %year is last four digits
      | 
      | last = get_param(sys,'LastModifiedDate');
      | if isempty(last)
      |     last = datestr(now,'yyyy');
      | else
      |     last = last(end-3:end);
      | end
      | 
      | if strcmp(first,last)
      |     fprintf('%s -- Copyright %s Nexteer',NxtrConf,first)
      | else
      |     fprintf('%s -- %s%s- %s Nexteer',NxtrConf,char(169),first,last)
      | end
  UpTh : Outport
  LowTh : Outport  Port=2
  wires:
  SysTqThdWide/1 -> UpTh/1
  Constant/1 -> LowTh/1

== system SF051A_SnsrOffsLrng/SnsrOffsLrng/SnsrOffsLrngPer2/Enable_Function/POC/Learn/BiasEstimation_ValidityCheck/HwTqAvrg_Check/Switch Case Action Subsystem2 ==
  SysTqThdWide : Inport
  Action Port : ActionPort  ActionType=case
  Constant : Constant  Value=ZERO_ULS_F32  OutDataTypeStr=single
      settings: AttributesFormatString=%<OutDataTypeStr>
  Gain : Gain  Gain=-1
  Subsystem5 : Subsystem  Description=|  mask(Copyright Information){none=on}
      | Copyright info block.                                               
      |                                                                     
      | Place copyright information at the top of every subsystem in design.
      mask prompts: none "No parameters"
      mask help: Place copyright information at the top of every subsystem in design.
      mask Display:
      | NxtrConf = 'Nexteer Confidential';
      | 
      | sys = bdroot; %handle for the current model ("system")
      | first = get_param(sys,'Created');
      | first = first(end-3:end);  %year is last four digits
      | 
      | last = get_param(sys,'LastModifiedDate');
      | if isempty(last)
      |     last = datestr(now,'yyyy');
      | else
      |     last = last(end-3:end);
      | end
      | 
      | if strcmp(first,last)
      |     fprintf('%s -- Copyright %s Nexteer',NxtrConf,first)
      | else
      |     fprintf('%s -- %s%s- %s Nexteer',NxtrConf,char(169),first,last)
      | end
  UpTh : Outport
  LowTh : Outport  Port=2
  wires:
  SysTqThdWide/1 -> Gain/1
  Gain/1 -> LowTh/1
  Constant/1 -> UpTh/1
